simulink model "AUV_ElectroMechanicsSSCPropeller"  (R2020a)
settings: Solver=ode23t  StartTime=0.0  StopTime=0.1  RelTol=1e-3
PreLoadFcn:
  | AUV_VehicleParameters;
libraries: fl_lib x13, nesl_utility x9, ee_lib x1, AUVPropulsionSSC_lib x1
settings Model: Creator=cosorio  LastModifiedBy=cosorio
settings DataIOCC: SaveOutput=off  DSMLogging=off  SaveTime=off  ReturnWorkspaceOutputs=off  SignalLoggingName=logsout_emSSCprop  ReturnWorkspaceOutputsName=out_ssc_pmsm_simplified
settings DebuggingCC: PregeneratedLibrarySubsystemCodeDiagnostic=none  ArithmeticOperatorsInVariantConditions=warning
settings SFSimCC: SimUseLocalCustomCode=off  CustomCodeUndefinedFunction=UseInterfaceOnly
settings RTWCC: RTWUseLocalCustomCode=off
settings SimscapeCC: SimscapeLogType=local  SimscapeLogName=simlog_emSSCprop  SimscapeLogLimitData=off

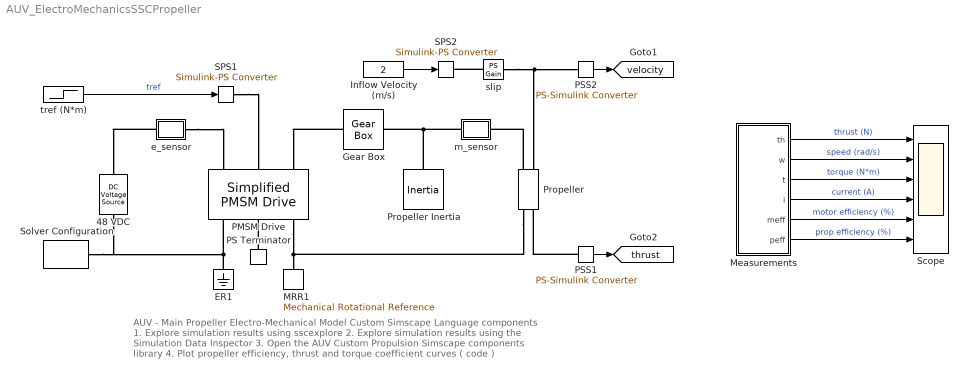
== system AUV_ElectroMechanicsSSCPropeller ==
  note: AUV - Main Propeller Electro-Mechanical Model
      | Custom Simscape Language components
      | 1. Explore simulation results using sscexplore
      | 2. Explore simulation results using the Simulation Data Inspector
      | 3. Open the AUV Custom Propulsion Simscape components library
      | 4. Plot propeller efficiency, thrust and torque coefficient curves ( code )
  48 VDC : fl_lib/Electrical/Electrical Sources/DC Voltage Source  v0=48 V
  ER1 : fl_lib/Electrical/Electrical Elements/Electrical Reference
      settings: SourceProductName=Foundation Library
  Gear Box : fl_lib/Mechanical/Mechanisms/Gear Box  ratio=6  t_in_specify=off  t_in_priority=None  t_in=0 N*m  t_in_nominal_specify=off  t_in_nominal_unit=N*m  t_in_nominal_value=1  t_out_specify=off  t_out_priority=None  t_out=0 N*m  t_out_nominal_specify=off  t_out_nominal_unit=N*m  t_out_nominal_value=1
  Inflow Velocity (m/s) : Constant  Value=2
  MRR1 : fl_lib/Mechanical/Rotational Elements/Mechanical Rotational Reference
  Measurements : Subsystem
  PMSM Drive : ee_lib/Electromechanical/Permanent Magnet/Simplified PMSM Drive  torque_speed_param=1  w_t=[0, 1200, 2950, 3600] rpm  T_t=[0.991, 0.980, 0.270, 0] N*m  torque_max=0.17 N*m  power_max=40 W  Tc=1/(2*pi*500) s  losses_param=1  eff=95  w_eff=7000 deg/s  T_eff=0.13 N*m  Piron=0 W  Pbase=0 W  w_eff_vec=[-8000, -4000, 0, 4000, 8000] rpm  T_eff_vec=[0, .03, .06, .09] N*m  v_eff_vec=[100, 250, 400] V  losses_mat=[1.49, 1.67, 2.21, 3.1; .42, .69, 1.14, 2.03; .06, .24, .78, 1.68; .42, .69, 1.14, 2.03; 1.49, 1.67, 2.21, 3.1] W  efficiency_mat=[95, 95, 95, 95; 95, 95, 95, 95; 95, 95, 95, 95; 95, 95, 95, 95; 95, 95, 95, 95]  losses_mat_3D=ones(5, 4, 3) W  efficiency_mat_3D=95 * ones(5, 4, 3)  Res=1.16 Ohm  J=30 g*cm^2  lam=1e-4 N*m/(rad/s)  speed0=0 deg/s  faulted_specify=off  faulted_priority=None  faulted=0  faulted_nominal_specify=off  faulted_nominal_unit=1  faulted_nominal_value=1  alpha=3.93e-3 1/K  Tmeas=25 degC  Tmeas2=125 degC  losses_mat_T2=[1.49, 1.74, 2.49, 3.74; .42, .67, 1.42, 2.67; .06, .31, 1.06, 2.31; .42, .67, 1.42, 2.67; 1.49, 1.74, 2.49, 3.74] W  efficiency_mat_T2=[95, 95, 95, 95; 95, 95, 95, 95; 95, 95, 95, 95; 95, 95, 95, 95; 95, 95, 95, 95]  losses_mat_3D_T2=ones(5, 4, 3) W  efficiency_mat_3D_T2=95 * ones(5, 4, 3)  thermal_mass=100 J/K  initial_temperature=25 degC  fault_condition=1  fault_threshold=0.5
      settings: SourceProductBaseCode=PS  LogSimulationData=on  InternalSimscapePortConfiguration="{\"Bottom\":[],\"Left\":[{\"id\":\"Vp\",\"label\":\"+\",\"type\":\"foundation.electrical.electrical\"},{\"id\":\"Tr\",\"label\":\"Tr\",\"type\":\"input\"},{\"id\":\"R\",\"label\":\"R\",\"type\":\"foundation.mechanical.rotational.rotational\"}],\"Right\":[{\"id\":\"Vm\",\"label\":\"-\",\"type\":\"foundation.electrical.electrical\"},{\"id\":\"Omega\",\"label\":\"w\",\"type\":\"output\"},{\"id\":\"C\",\"label\":\"C\",\"type\":\"foundation.mechanical.rotational.rotational\"}],\"Top\":[]}"
  PS Terminator : fl_lib/Physical Signals/Sinks/PS Terminator
  PSS1 : nesl_utility/PS-Simulink Converter  PhysicalDomain=network_engine_domain  SubClassName=ps_output  LeftPortType=input  RightPortType=output  PseudoPeriodic=off  Frequencies=[]  Unit=N  AffineConversion=off
  PSS2 : nesl_utility/PS-Simulink Converter  PhysicalDomain=network_engine_domain  SubClassName=ps_output  LeftPortType=input  RightPortType=output  PseudoPeriodic=off  Frequencies=[]  Unit=m/s  AffineConversion=off
  Propeller : AUVPropulsionSSC_lib/Propeller  D=0.3 m  ktPoly="[0.0408   -0.2896   -0.1114    0.5420]"  kqPoly="[-0.0157   -0.0084   -0.0283    0.0947]"  rho=1027.3 kg/m^3  w_specify=off  w_priority=None  w=0 rad/s  w_nominal_specify=off  w_nominal_unit=rad/s  w_nominal_value=1  t_specify=off  t_priority=None  t=0 N*m  t_nominal_specify=off  t_nominal_unit=N*m  t_nominal_value=1
      settings: InternalSimscapePortConfiguration="{\"Bottom\":[],\"Left\":[{\"id\":\"Va\",\"label\":\"Va\",\"type\":\"input\"},{\"id\":\"R\",\"label\":\"R\",\"type\":\"foundation.mechanical.rotational.rotational\"}],\"Right\":[{\"id\":\"Thrust\",\"label\":\"Th\",\"type\":\"output\"},{\"id\":\"C\",\"label\":\"C\",\"type\":\"foundation.mechanical.rotational.rotational\"}],\"Top\":[]}"
  Propeller Inertia : fl_lib/Mechanical/Rotational Elements/Inertia  inertia=0.00015 kg*m^2  w_specify=off  w_priority=High  w=0 rad/s  w_nominal_specify=off  w_nominal_unit=rad/s  w_nominal_value=1  t_specify=off  t_priority=None  t=0 N*m  t_nominal_specify=off  t_nominal_unit=N*m  t_nominal_value=1
      settings: LogSimulationData=on
  SPS1 : nesl_utility/Simulink-PS Converter  PhysicalDomain=network_engine_domain  SubClassName=ps_input  LeftPortType=input  RightPortType=output  PseudoPeriodic=off  Frequencies=[]  NoiseDistribution=none  NoiseParameters=[]  Unit=N*m  AffineConversion=off  FilteringAndDerivatives=provide  SimscapeFilterOrder=1  InputFilterTimeConstant=0.001  UdotUserProvided=0
  SPS2 : nesl_utility/Simulink-PS Converter  PhysicalDomain=network_engine_domain  SubClassName=ps_input  LeftPortType=input  RightPortType=output  PseudoPeriodic=off  Frequencies=[]  NoiseDistribution=none  NoiseParameters=[]  Unit=m/s  AffineConversion=off  FilteringAndDerivatives=provide  SimscapeFilterOrder=1  InputFilterTimeConstant=0.001  UdotUserProvided=0
  Scope : Scope  NumInputPorts=6
  Solver Configuration : nesl_utility/Solver Configuration  PhysicalDomain=network_engine_domain  SubClassName=solver  LeftPortType=input  RightPortType=generic  Tones=[]  Harmonics=[]  SimulateNoise=off  Profile=off  UseLocalSampling=off  EnableSwitchedLinearOptims=on  FrequencyDomain=off  UseCCode=off  RelTol=0.001  AbsTol=1e-06  MinStep=1e-09  ToWorkspace=off  RevertToSquareIcSolve=off  NumHomotopyIterations=100  PhasorMode=off  PhasorModeNumHarmonics=1  DoDC=off  ResidualTolerance=1e-09  UseLocalSolver=off  LocalSolverChoice=NE_PARTITIONING_ADVANCER  LocalSolverSampleTime=1e-5  DoFixedCost=off  MaxNonlinIter=3  MaxModeIter=2  LinearAlgebra=Sparse  EquationFormulation=NE_TIME_EF  DelaysMemoryBudget=1024  AutomaticFiltering=on  FilteringTimeConstant=0.001  PartitionStorageMethod=AS_NEEDED  PartitionMemoryBudget=1024  PartitionMethod=FAST
  e_sensor : Subsystem
  m_sensor : Subsystem
  slip : fl_lib/Physical Signals/Functions/PS Gain  gain=1
  tref (N*m) : Step  Time=0.05  Before=0.25  After=0.5  SampleTime=0
  tag scope: thrust=global, velocity=global
  wires:
  tref (N*m)/1 -> SPS1/1  "tref"
  Measurements/2(w) -> Scope/2  "speed (rad/s)"
  Measurements/3(t) -> Scope/3  "torque (N*m)"
  Measurements/4(i) -> Scope/4  "current (A)"
  Measurements/5(meff) -> Scope/5  "motor efficiency (%)"
  PSS1/1 -> [thrust]
  Measurements/1(th) -> Scope/1  "thrust (N)"
  Inflow Velocity (m/s)/1 -> SPS2/1
  PSS2/1 -> [velocity]
  Measurements/6(peff) -> Scope/6  "prop efficiency (%)"
  connections:
  PMSM Drive/RConn3 -- Propeller/RConn2 -- MRR1/LConn1
  ER1/LConn1 -- 48 VDC/RConn1 -- Solver Configuration/RConn1 -- PMSM Drive/RConn1
  SPS1/RConn1 -- PMSM Drive/LConn2
  Gear Box/LConn1 -- PMSM Drive/LConn3
  PS Terminator/LConn1 -- PMSM Drive/RConn2
  e_sensor/RConn1 -- PMSM Drive/LConn1
  e_sensor/LConn1 -- 48 VDC/LConn1
  Propeller/LConn2 -- m_sensor/RConn1
  m_sensor/LConn1 -- Gear Box/RConn1 -- Propeller Inertia/LConn1
  PSS1/LConn1 -- Propeller/RConn1
  slip/LConn1 -- SPS2/RConn1
  slip/RConn1 -- PSS2/LConn1 -- Propeller/LConn1

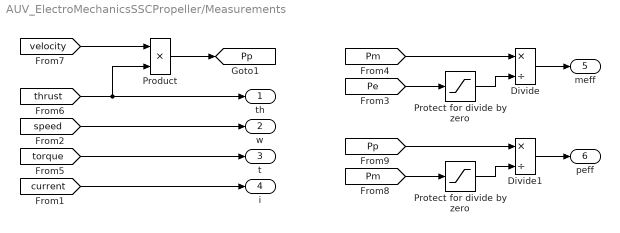
== system AUV_ElectroMechanicsSSCPropeller/Measurements ==
  Divide : Product  Inputs=*/
  Divide1 : Product  Inputs=*/
  Product : Product
  Protect for divide by zero : Saturate  UpperLimit=inf  LowerLimit=1e-3
  "Protect for divide by zero " : Saturate  UpperLimit=inf  LowerLimit=1e-3
  th : Outport
  w : Outport  Port=2
  t : Outport  Port=3
  i : Outport  Port=4
  meff : Outport  Port=5
  peff : Outport  Port=6
  tag scope: Pp=global
  wires:
  Divide/1 -> meff/1
  [current] -> i/1
  [Pe] -> Protect for divide by zero/1
  [torque] -> t/1
  [speed] -> w/1
  [Pm] -> Divide/1
  Protect for divide by zero/1 -> Divide/2
  [thrust] -> th/1, Product/2
  [velocity] -> Product/1
  Product/1 -> [Pp]
  "Protect for divide by zero "/1 -> Divide1/2
  [Pp] -> Divide1/1
  [Pm] -> "Protect for divide by zero "/1
  Divide1/1 -> peff/1

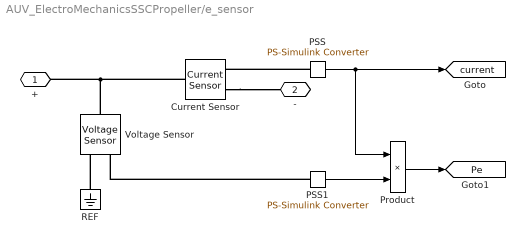
== system AUV_ElectroMechanicsSSCPropeller/e_sensor ==
  Current Sensor : fl_lib/Electrical/Electrical Sensors/Current Sensor
  PSS : nesl_utility/PS-Simulink Converter  PhysicalDomain=network_engine_domain  SubClassName=ps_output  LeftPortType=input  RightPortType=output  PseudoPeriodic=off  Frequencies=[]  Unit=A  AffineConversion=off
  PSS1 : nesl_utility/PS-Simulink Converter  PhysicalDomain=network_engine_domain  SubClassName=ps_output  LeftPortType=input  RightPortType=output  PseudoPeriodic=off  Frequencies=[]  Unit=V  AffineConversion=off
  Product : Product
  REF : fl_lib/Electrical/Electrical Elements/Electrical Reference
  Voltage Sensor : fl_lib/Electrical/Electrical Sensors/Voltage Sensor
  + : PMIOPort  Side=Left
  - : PMIOPort  Port=2  Side=Right
  tag scope: Pe=global, current=global
  wires:
  PSS/1 -> [current], Product/1
  PSS1/1 -> Product/2
  Product/1 -> [Pe]
  connections:
  Current Sensor/LConn1 -- Voltage Sensor/LConn1 -- +/RConn1
  Current Sensor/RConn2 -- -/RConn1
  PSS/LConn1 -- Current Sensor/RConn1
  REF/LConn1 -- Voltage Sensor/RConn2
  PSS1/LConn1 -- Voltage Sensor/RConn1

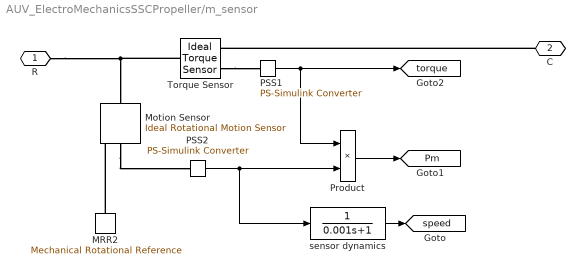
== system AUV_ElectroMechanicsSSCPropeller/m_sensor ==
  MRR2 : fl_lib/Mechanical/Rotational Elements/Mechanical Rotational Reference
  Motion Sensor : fl_lib/Mechanical/Mechanical Sensors/Ideal Rotational Motion Sensor  wrap_angle=simscape.enum.onoff.off  offset=0 rad
  PSS1 : nesl_utility/PS-Simulink Converter  PhysicalDomain=network_engine_domain  SubClassName=ps_output  LeftPortType=input  RightPortType=output  PseudoPeriodic=off  Frequencies=[]  Unit=N*m  AffineConversion=off
  PSS2 : nesl_utility/PS-Simulink Converter  PhysicalDomain=network_engine_domain  SubClassName=ps_output  LeftPortType=input  RightPortType=output  PseudoPeriodic=off  Frequencies=[]  Unit=rad/s  AffineConversion=off
  Product : Product
  Torque Sensor : fl_lib/Mechanical/Mechanical Sensors/Ideal Torque Sensor
  sensor dynamics : TransferFcn  Denominator=[0.001 1]
  R : PMIOPort  Side=Left
  C : PMIOPort  Port=2  Side=Right
  tag scope: Pm=global, speed=global, torque=global
  wires:
  PSS2/1 -> Product/2, sensor dynamics/1
  sensor dynamics/1 -> [speed]
  Product/1 -> [Pm]
  PSS1/1 -> Product/1, [torque]
  connections:
  MRR2/LConn1 -- Motion Sensor/RConn1
  R/RConn1 -- Torque Sensor/LConn1 -- Motion Sensor/LConn1
  Motion Sensor/RConn2 -- PSS2/LConn1
  C/RConn1 -- Torque Sensor/RConn1
  Torque Sensor/RConn2 -- PSS1/LConn1
